simulink model "firstExerciseSecondorderMovingAverage"  (R2024b)
settings: Solver=VariableStepAuto  StartTime=0.0  StopTime=10.0  RelTol=1e-3
settings Model: Creator=rasm2  LastModifiedBy=rasm2

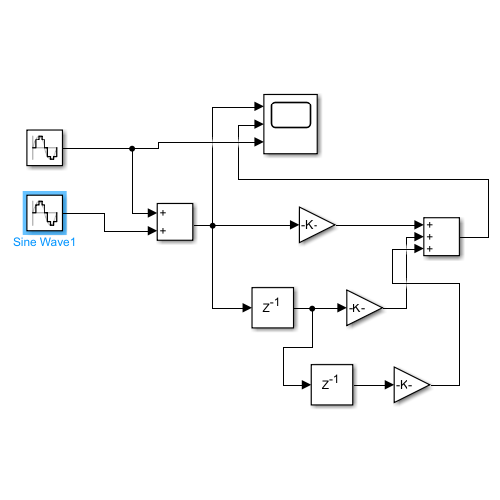
[thumbnail: Simulink's stored preview of the top-level diagram]
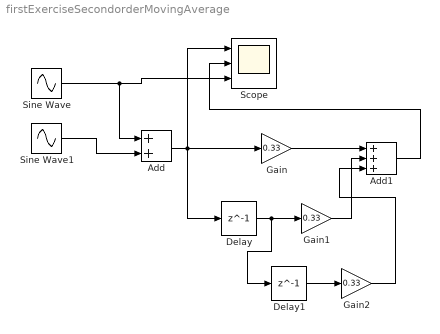
== system firstExerciseSecondorderMovingAverage ==
  Add : Sum
  Add1 : Sum  Inputs=+++
  Delay : Delay  DelayLength=1
  Delay1 : Delay  DelayLength=1
  Gain : Gain  Gain=0.33
  Gain1 : Gain  Gain=0.33
  Gain2 : Gain  Gain=0.33
  Scope : Scope  NumInputPorts=3
  Sine Wave : Sin  Tag=base signal  Amplitude=10  SampleTime=0.2
  Sine Wave1 : Sin  Amplitude=10  Frequency=2  SampleTime=0.2
  wires:
  Sine Wave1/1 -> Add/2
  Sine Wave/1 -> Scope/3, Add/1
  Add/1 -> Scope/1, Delay/1, Gain/1
  Delay/1 -> Delay1/1, Gain1/1
  Gain/1 -> Add1/1
  Gain1/1 -> Add1/2
  Add1/1 -> Scope/2
  Delay1/1 -> Gain2/1
  Gain2/1 -> Add1/3
